simulink model "Human_in_Loop"  (R2017b)
settings: Solver=ode1  StartTime=0.0  StopTime=Inf  FixedStep=0.0002  RelTol=1e-3
PostLoadFcn:
  | , if any(exist('dsrtsu_mdlpostloadfcn', 'file') == [2, 3, 6]), try dsrtsu_mdlpostloadfcn('Execute', bdroot); catch fprintf('Error in PostLoadFcn (dsrtsu_mdlpostloadfcn) for model "%s":\n %s\n', bdroot, lasterr); end, end,
libraries: rti1202lib_dio_class1 x4, rti1202serlib x3, rtiemclib x2, rti1202lib_dac_class1 x1, simulink x1, rti1202lib_adc_class1 x1, rtitasklib x1
(part 2 of 2)

== system Human_in_Loop/Sensor Data/Cosmed/COSMED ==
  time : Inport
  count : Inport  Port=2
  DS1202SER_INT_C1_I1 : rti1202serlib/DS1202SER_INT_C1_I1  Reserved1=[]  Reserved2=[]  Reserved3=[]  Reserved4=[]  DSProperties=struct('RTI',struct('IOBoardType',{{'DS1202','SER'}},'SlaveProcessor','NONE','Version',uint32(3),'BlockType',struct('isSLSource',uint8(1),'isSLSink',uint8(0),'isHWSource',uint8(0),'isHWSink',uint8(0),'isSetup',uint8(0),'isInline',uint8(1),'isNonInline',uint8(0),'isInterrupt',uint8(1),'isChannelwise',uint8(1)),'UnitType','GENSER','Identifier','SERINT','DialogType','ML','BlockSet','NONE','RelationId',struct('TH',struct('BlockId','HWINT'))))  RTIBlockInterface=struct('BlockDisplay',{{['DS1202 SER Interrupt\n Channel 1\nReceive Interrupt'],'center'}},'BlockName',struct('Token',{{'DS1202SER_INT_C','_I'}},'BlockParam',{{'ChannelNo','IntType'}}),'OutputPortsWidth',int32(1),'OutputPortsActive',1,'OutputPortsName',{{[' ']}},'IconTransparency','off','ParameterTunableNames',{{}},'InitLevel',3,'DialogFcn','guigenserserint','MaskDescription',['To make the interrupts of the UART serial interface available as trigger source.'],'FunctionCall',uint32(0),'Options',{{'SS_OPTION_FORCE_NONINLINED_FCNCALL','SS_OPTION_ASYNCHRONOUS_INTERRUPT'}})  RTIBlockParameters=struct('ThIntNo',{{'UART_EVENTS','OFF',[]}},'ThSubIntNo',{{0,'ON',[0 4]}},'ThSrcSgnName',{{['UART Ch1 RX SW FIFO interrupt'],'OFF',[]}},'TLCFileName',{{'rti_hwinterrupt','OFF',[]}},'BoardNo',{{1,'ON',[1 1]}},'ChannelNo',{{1,'ON',[1 2]}},'ChannelNumOf',{{2,'OFF',[]}},'ThBlk',{{['struct(''blkh'',[''Human_in_Loop/Sensor Data/Cosmed/COSMED/DS1202SER_INT_C1_I1''],''srcId'',''UART_EVENTS_CH1_INT0'',''srcSgnId'',''UART_EVENTS_CH1_INT0'',''intervalTmrBlockId'',[],''srcSgnName'',[''UART Ch1 RX SW FIFO interrupt''],''srcCpuId'','''',''isSrcCpu'',1,''isTargetCpu'',1,''srcOnMasterCpu'',1,''boardType'','''',''boardTypeNo'','''',''boardNo'',1,''intNo'',''UART_EVENTS'',''subIntNo'',0,''period'',0,''entryPoint'',''rti_UART_EVENTS_CH1_INT0'',''blockName'',''DS1202SER_INT_C1_I1'',''taskNameDisplayExt'','''',''taskType'',''HWINT'',''groupId'',''SERINT'',''hookFcn'',''NULL'',''isTimerTaskSrc'',0,''service'','''',''mpBlkId'','''',''taskPriorityPreConfig'',''none'',''taskPriority'',-1,''taskSortWeighting'',[],''taskSchedulingPolicy'',''FCFS'',''taskOvrPreConfig'',''none'',''taskOvrStrategy'',1,''taskOvrQueueSize'',1,''taskVisibility'',''on'',''taskGroupId'','''',''taskGroupDisplayOrder'',[],''serviceDynamicGen'',0,''disableCodeGen'',0,''boardBase'',''IOLIB_SPEC_INT_UART(1)'',''noBoardBase'','''')'],'OFF',[]}},'IntType',{{1,'ON',[1 4]}},'ReceiveIntLevelFifo',{{'1','OFF',[]}},'IntTypeMacro',{{'DSSER_TRIGGER_LEVEL_SUBINT_MASK','OFF',[]}},'FifoSizeDefault',{{64,'OFF',[]}})  RTISFcnParameters=struct('BoardNo','double','ChannelNo','double','ThIntNo','double','ThSubIntNo','double','ThBlk','struct','IntType','double','ReceiveIntLevelFifo','double','TLCFileName','char','IntTypeMacro','char')  RTIBlockParaDefault=struct('ThIntNo',1,'ThSubIntNo',0,'ThSrcSgnName',['RX SW FIFO interrupt'],'TLCFileName','rti_hwinterrupt','BoardNo',1,'ChannelNo',1,'ChannelNumOf',2,'ThBlk',['struct(''srcSgnId'', '''')'],'IntType',1,'ReceiveIntLevelFifo',1,'IntTypeMacro','DSSER_TRIGGER_LEVEL_SUBINT_MASK','FifoSizeDefault',64)
  DS1202SER_SETUP_C1 : rti1202serlib/DS1202SER_SETUP_C1  Reserved1=[]  Reserved2=[]  Reserved3=[]  Reserved4=[]  DSProperties=struct('RTI',struct('Version',uint32(2),'IOBoardType',{{'DS1202','SER'}},'SlaveProcessor','NONE','BlockType',struct('isSLSource',uint8(0),'isSLSink',uint8(0),'isHWSource',uint8(0),'isHWSink',uint8(0),'isSetup',uint8(1),'isInline',uint8(1),'isNonInline',uint8(0),'isInterrupt',uint8(0),'isChannelwise',uint8(1)),'UnitType','GENSER','Identifier','SETUP','DialogType','ML','BlockSet','NONE'))  RTIBlockInterface=struct('BlockName',struct('Token',{{'DS1202SER_SETUP_C'}},'BlockParam',{{'ChannelNo'}}),'BlockDisplay',{{['Serial Setup'],'center'}},'IconTransparency','off','ParameterTunableNames',{{}},'InitLevel',1,'DialogFcn','guigensersetup','MaskDescription',['To set the global specifications for the UART interface.'])  RTIBlockParameters=struct('ParityMode',{{1,'OFF',[1 5]}},'TransceiverMode',{{[1;1],'OFF',[]}},'QuartzFrequency',{{'160000000','OFF',[]}},'BoardNo',{{1,'ON',[1 1]}},'ChannelNo',{{1,'ON',[1 2]}},'ChannelNumOf',{{2,'OFF',[]}},'BaudRate',{{'115200','OFF',[]}},'DataBitsNumOf',{{4,'OFF',[1 4]}},'StopBitsNumOf',{{1,'OFF',[1 3]}},'ReceiveIntLevelUart',{{4,'OFF',[1 4]}},'AutoflowMode',{{0,'OFF',[]}},'FifoSize',{{'256','OFF',[]}},'ReceiveIntLevelFifo',{{0,'OFF',[]}},'FifoOverrunMode',{{1,'OFF',[]}},'FifoBlockSize',{{'0','OFF',[]}},'TermMode',{{1,'OFF',[]}},'TLCFileName',{{'rtigensersetup','OFF',[]}})  RTISFcnParameters=struct('BoardNo','double','ChannelNo','double','ChannelNumOf','double','BaudRate','double','DataBitsNumOf','double','StopBitsNumOf','double','ParityMode','double','TransceiverMode','double','ReceiveIntLevelUart','double','AutoflowMode','double','FifoSize','double','ReceiveIntLevelFifo','double','FifoBlockSize','double','TermMode','double','QuartzFrequency','double','TLCFileName','char')  RTIBlockParaDefault=struct('ParityMode',1,'TransceiverMode',[1;1],'QuartzFrequency',160000000,'BoardNo',1,'ChannelNo',1,'ChannelNumOf',2,'BaudRate',115200,'DataBitsNumOf',4,'StopBitsNumOf',1,'ReceiveIntLevelUart',4,'AutoflowMode',0,'FifoSize',64,'ReceiveIntLevelFifo',0,'FifoOverrunMode',1,'FifoBlockSize',0,'TermMode',1,'TLCFileName','rtigensersetup')
  Serial Decoding System : Subsystem
  E : Outport
  wires:
  DS1202SER_INT_C1_I1/1 -> Serial Decoding System/Trigger
  Serial Decoding System/1(E) -> E/1
  time/1 -> Serial Decoding System/1(time)
  count/1 -> Serial Decoding System/2(count)

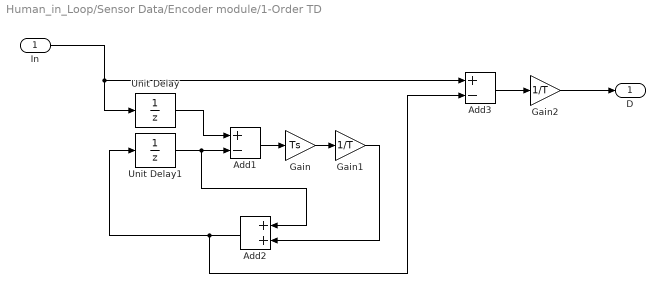
== system Human_in_Loop/Sensor Data/Encoder module/1-Order TD ==
  In : Inport
  Add1 : Sum  Inputs=+-
  Add2 : Sum
  Add3 : Sum  Inputs=+-
  Gain : Gain  Gain=Ts
  Gain1 : Gain  Gain=1/T
  Gain2 : Gain  Gain=1/T
  Unit Delay : UnitDelay  SampleTime=-1
  Unit Delay1 : UnitDelay  SampleTime=-1
  D : Outport
  wires:
  Unit Delay/1 -> Add1/1
  Add2/1 -> Add3/2, Unit Delay1/1
  Unit Delay1/1 -> Add2/1, Add1/2
  Add1/1 -> Gain/1
  Gain/1 -> Gain1/1
  Gain1/1 -> Add2/2
  In/1 -> Unit Delay/1, Add3/1
  Add3/1 -> Gain2/1
  Gain2/1 -> D/1

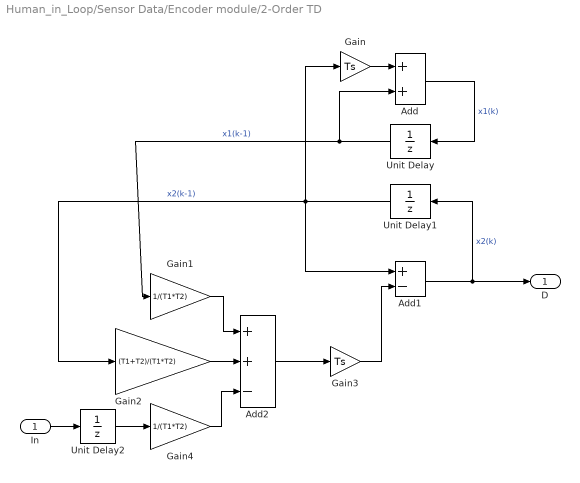
== system Human_in_Loop/Sensor Data/Encoder module/2-Order TD ==
  In : Inport
  Add : Sum
  Add1 : Sum  Inputs=+-
  Add2 : Sum  Inputs=++-
  Gain : Gain  Gain=Ts
  Gain1 : Gain  Gain=1/(T1*T2)
  Gain2 : Gain  Gain=(T1+T2)/(T1*T2)
  Gain3 : Gain  Gain=Ts
  Gain4 : Gain  Gain=1/(T1*T2)
  Unit Delay : UnitDelay  SampleTime=-1
  Unit Delay1 : UnitDelay  SampleTime=-1
  Unit Delay2 : UnitDelay  SampleTime=-1
  D : Outport
  wires:
  Unit Delay1/1 -> Gain2/1, Gain/1, Add1/1  "x2(k-1)"
  Gain/1 -> Add/1
  Add/1 -> Unit Delay/1  "x1(k)"
  Unit Delay/1 -> Gain1/1, Add/2  "x1(k-1)"
  Add1/1 -> D/1, Unit Delay1/1  "x2(k)"
  Gain1/1 -> Add2/1
  In/1 -> Unit Delay2/1
  Gain2/1 -> Add2/2
  Add2/1 -> Gain3/1
  Gain3/1 -> Add1/2
  Unit Delay2/1 -> Gain4/1
  Gain4/1 -> Add2/3

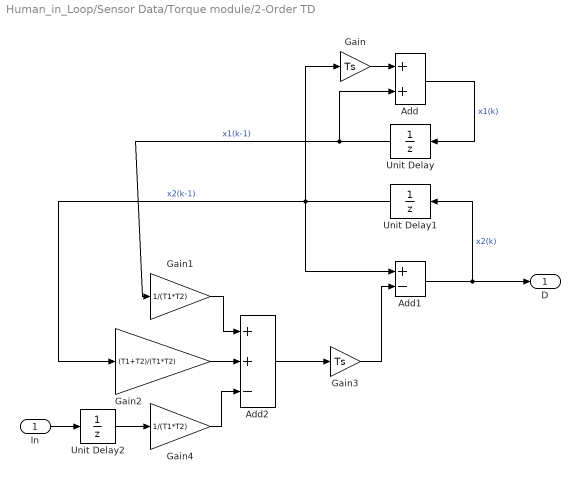
== system Human_in_Loop/Sensor Data/Torque module/2-Order TD ==
  In : Inport
  Add : Sum
  Add1 : Sum  Inputs=+-
  Add2 : Sum  Inputs=++-
  Gain : Gain  Gain=Ts
  Gain1 : Gain  Gain=1/(T1*T2)
  Gain2 : Gain  Gain=(T1+T2)/(T1*T2)
  Gain3 : Gain  Gain=Ts
  Gain4 : Gain  Gain=1/(T1*T2)
  Unit Delay : UnitDelay  SampleTime=-1
  Unit Delay1 : UnitDelay  SampleTime=-1
  Unit Delay2 : UnitDelay  SampleTime=-1
  D : Outport
  wires:
  Unit Delay1/1 -> Gain2/1, Gain/1, Add1/1  "x2(k-1)"
  Gain/1 -> Add/1
  Add/1 -> Unit Delay/1  "x1(k)"
  Unit Delay/1 -> Gain1/1, Add/2  "x1(k-1)"
  Add1/1 -> D/1, Unit Delay1/1  "x2(k)"
  Gain1/1 -> Add2/1
  In/1 -> Unit Delay2/1
  Gain2/1 -> Add2/2
  Add2/1 -> Gain3/1
  Gain3/1 -> Add1/2
  Unit Delay2/1 -> Gain4/1
  Gain4/1 -> Add2/3

== system Human_in_Loop/RTI Data/RTI Data Store/RTI Data Store/RTI Data Store ==
  RTI Data Store : Subsystem  mask(RTI_DATA_STORE){}
      mask help:
      | RTI Data Store Block. This block is used by RTI to store internal model dependent data. Deleting this block will result in data loss.
      |
      | NEVER DELETE, COPY, OR MODIFY THIS BLOCK!
      mask Help:
      | RTI Data Store Block. This block is used by RTI to store internal model dependent data. Deleting this block will result in data loss.
      | 
      | NEVER DELETE, COPY, OR MODIFY THIS BLOCK!
      mask Display: text(0.5, 0.5, ' ', 'HorizontalAlignment', 'center');

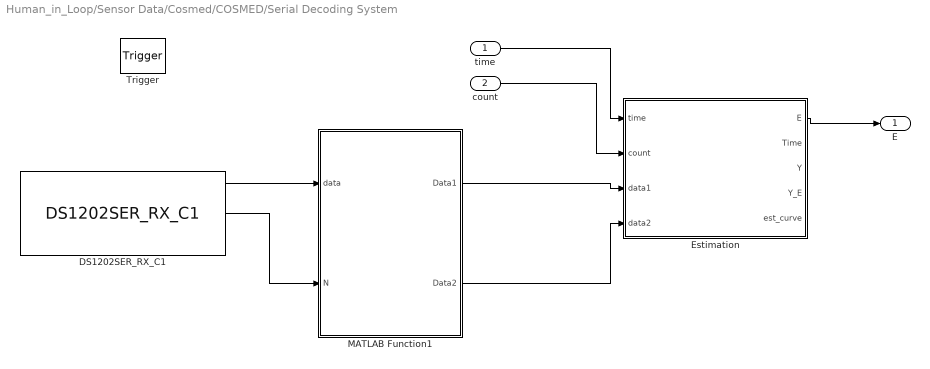
== system Human_in_Loop/Sensor Data/Cosmed/COSMED/Serial Decoding System ==
  time : Inport
  count : Inport  Port=2
  Trigger : TriggerPort  TriggerType=function-call  VariantControl=(inherit)
  DS1202SER_RX_C1 : rti1202serlib/DS1202SER_RX_C1  Reserved1=[]  Reserved2=[]  Reserved3=[]  Reserved4=[]  DSProperties=struct('RTI',struct('IOBoardType',{{'DS1202','SER'}},'SlaveProcessor','NONE','Version',uint32(1),'BlockType',struct('isSLSource',uint8(1),'isSLSink',uint8(1),'isHWSource',uint8(0),'isHWSink',uint8(1),'isSetup',uint8(0),'isInline',uint8(1),'isNonInline',uint8(0),'isInterrupt',uint8(0),'isChannelwise',uint8(1)),'UnitType','GENSER','Identifier','RECEIVE','DialogType','ML','BlockSet','NONE'))  RTIBlockInterface=struct('BlockName',struct('Token',{{'DS1202SER_RX_C'}},'BlockParam',{{'ChannelNo'}}),'InputPortsWidth',int32(1),'InputPortsActive',0,'InputPortsDataType',{{'SS_UINT32'}},'InputPortsName',{{'NumBytes'}},'OutputPortsWidth',int32([16 1 1]),'OutputPortsActive',[1 1 1],'OutputPortsDataType',{{'SS_UINT8','SS_UINT32','SS_INT32'}},'OutputPortsName',{{'RXBytes','NumRXBytes','Status'}},'BlockDisplay',{{['Serial Receive'],'center'}},'IconTransparency','on','ParameterTunableNames',{{}},'InitLevel',2,'DialogFcn','guigenserreceive','MaskDescription',['To read data from the UART SW FIFO.'])  RTIBlockParameters=struct('BoardNo',{{1,'ON',[1 1]}},'ChannelNo',{{1,'ON',[1 2]}},'ChannelNumOf',{{2,'OFF',[]}},'ReceptionDataMode',{{1,'OFF',[]}},'ParamTunableMode',{{2,'OFF',[]}},'BytesRefNumOfT',{{'1','OFF',[1 inf]}},'BytesRefNumOfNT',{{'16','OFF',[1 inf]}},'BytesRefNumOfMax',{{'1','OFF',[1 inf]}},'BytesRefNumOfMode',{{0,'OFF',[]}},'BytesActNumOfMode',{{1,'OFF',[]}},'ReceptionStatusMode',{{1,'OFF',[]}},'FifoSizeDefault',{{64,'OFF',[]}},'TLCFileName',{{'rtigenserreceive','OFF',[]}})  RTISFcnParameters=struct('BoardNo','double','ChannelNo','double','ChannelNumOf','double','ReceptionDataMode','double','ParamTunableMode','double','BytesRefNumOfT','double','BytesRefNumOfNT','double','BytesRefNumOfMax','double','BytesRefNumOfMode','double','BytesActNumOfMode','double','ReceptionStatusMode','double','TLCFileName','char')  RTIBlockParaDefault=struct('BoardNo',1,'ChannelNo',1,'ChannelNumOf',2,'ReceptionDataMode',1,'ParamTunableMode',1,'BytesRefNumOfT',1,'BytesRefNumOfNT',1,'BytesRefNumOfMax',1,'BytesRefNumOfMode',0,'BytesActNumOfMode',1,'ReceptionStatusMode',1,'FifoSizeDefault',64,'TLCFileName','rtigenserreceive')
  Estimation : MATLAB Function  TreatAsAtomicUnit=on
  MATLAB Function1 : MATLAB Function  TreatAsAtomicUnit=on
  E : Outport
  wires:
  DS1202SER_RX_C1/2 -> MATLAB Function1/2(N)
  MATLAB Function1/1(Data1) -> Estimation/3(data1)
  DS1202SER_RX_C1/1 -> MATLAB Function1/1(data)
  time/1 -> Estimation/1(time)
  count/1 -> Estimation/2(count)
  Estimation/1(E) -> E/1
  MATLAB Function1/2(Data2) -> Estimation/4(data2)

== system Human_in_Loop/RTI Data/RTI Data Store/RTI Data Store/RTI Data Store/RTI Data Store ==

== matlab function Human_in_Loop/Sensor Data/Encoder module/Data process ==
  data: encoder input; angle output; BT_RESET_ANKLE parameter boolean
function angle = process(encoder, BT_RESET_ANKLE)

    persistent angle_zero;
    if isempty(angle_zero)
        angle_zero = 0;
    end

    if BT_RESET_ANKLE == 1
        angle_zero = encoder;
    end

    angle = encoder - angle_zero;
end

== matlab function Human_in_Loop/Sensor Data/Encoder module/Data process1 ==
  data: encoder input; BT_RESET_MOTOR parameter boolean; angle output
function angle = process(encoder, BT_RESET_MOTOR)

    persistent angle_zero;
    if isempty(angle_zero)
        angle_zero = 0;
    end

    if BT_RESET_MOTOR == 1
        angle_zero = encoder;
    end

    angle = encoder - angle_zero;
    
end

== matlab function Human_in_Loop/Sensor Data/Encoder module/Mux ==
  data: x1 input; x output; x2 input
function x = mux(x1,x2)

x = [x1 x2];

== matlab function Human_in_Loop/Sensor Data/Torque module/Data process ==
  data: vol input; torque output; load_vol_gain parameter double; load_vol_offset parameter double; BT_RESET_TORQUE parameter boolean
function torque = process(vol, load_vol_gain, load_vol_offset, BT_RESET_TORQUE)
%% 功能：电压-力矩转换与力矩归零

    persistent torque_zero;
    if isempty(torque_zero)
        torque_zero = 0;
    end

    %%% 力矩归零
    if BT_RESET_TORQUE == 1
        torque_zero = vol*load_vol_gain + load_vol_offset;
    end

    torque = vol*load_vol_gain + load_vol_offset - torque_zero;

end

== matlab function Human_in_Loop/Sensor Data/Encoder module/Mux1 ==
  data: x1 input; x output; x2 input; x3 input
function x = mux(x1,x2,x3)

x = [x1 x2 x3];

== matlab function Human_in_Loop/Sensor Data/Encoder module/Mux2 ==
  data: x1 input; x output; x2 input; x3 input
function x = mux(x1,x2,x3)

x = [x1 x2 x3];

== matlab function Human_in_Loop/Sensor Data/FootSwitch module/FootSwitch Filter ==
  data: signal input; state output
function state = filter(signal)

%% 对足底开关信号进行滤波
% 滤波原则：上升沿无滤波，下降沿消抖滤波

Ts = 0.0002;
persistent foot_state;
persistent filter_time;
if isempty(foot_state)
    foot_state = 0;
    filter_time = 0;
end

if foot_state == 0
    if signal == 1
        foot_state = 1;
    else
        foot_state = 0;
    end
else
    if signal == 1
        foot_state = 1;
    else
        filter_time = filter_time + Ts;
        if filter_time > 0.1
            filter_time = 0;
            foot_state = 0;
        end
    end
end
   
state = foot_state;

end

== matlab function Human_in_Loop/Parameter Module/Control Parameter/Mux1 ==
  data: x1 input; x output; x2 input; x3 input; x4 input; x5 input
function x = mux(x1,x2,x3,x4,x5)

x = [x1 x2 x3 x4 x5];

== matlab function Human_in_Loop/Parameter Module/Torque Parameter/Mux1 ==
  data: x1 input; x output; x2 input; x3 input; x4 input
function x = mux(x1,x2,x3,x4)

x = [x1 x2 x3,x4];

== matlab function Human_in_Loop/State Module/State Machine ==
  data: mode output; footswitch input; state output; BT_RUN parameter boolean; BT_SLACK parameter boolean; BT_IDLE parameter boolean; BT_ERROR parameter boolean; stride_time output; BT_CALIB parameter boolean; stride_timer output
function [mode,state,stride_time,stride_timer] = StateMechine(footswitch, BT_RUN, BT_SLACK, BT_IDLE, BT_ERROR, BT_CALIB)

%% 定义寄存变量
persistent reg_stride_time;
persistent reg_stride_time_count;
persistent reg_mode;
persistent reg_state;
persistent bt_run;
persistent reg_last_switch;
if isempty(reg_stride_time)
    reg_stride_time = 1;
    reg_stride_time_count = 0;
    reg_mode = 1;
    reg_state = 1;
    bt_run = 0;
    reg_last_switch = 1;
end

%% 参数定义
Ts = 0.0002;
PP_StandSwing = 0.6;
max_stride_time = 1.5;
min_sride_time = 0.5;

%% 模式说明
IDLE_MODE  = 1;
RUN_MODE   = 2;
SLACK_MODE = 3;
CALIB_MODE = 4;
ERROR_MODE = 0;

%% 模式转换
if BT_RUN == 1
    bt_run = 1;
end
if BT_CALIB == 1
    reg_mode = CALIB_MODE;
end
if BT_SLACK == 1
    reg_mode = SLACK_MODE;
end
if BT_IDLE == 1
    reg_mode = IDLE_MODE;
end
if BT_ERROR == 1
    reg_mode = ERROR_MODE;
end
% 运行模式在swing->stance时切换
if bt_run == 1 && reg_last_switch == 0 && footswitch == 1
    reg_mode = RUN_MODE;
    bt_run = 0;
end
        
if reg_mode == RUN_MODE || reg_mode == IDLE_MODE
    if reg_last_switch == 0 && footswitch == 1
        reg_state = 1;
        reg_stride_time = 0.618*reg_stride_time + 0.382*reg_stride_time_count;
        reg_stride_time_count = 0;
    elseif reg_state ==1 && reg_stride_time_count > PP_StandSwing * reg_stride_time
        reg_state = 0;
        reg_stride_time_count = reg_stride_time_count + Ts;
    else
        reg_stride_time_count = reg_stride_time_count + Ts;
    end
end

reg_last_switch = footswitch;
if reg_stride_time > max_stride_time
    reg_stride_time = max_stride_time;
elseif reg_stride_time < min_sride_time
    reg_stride_time = min_sride_time;
end

mode = reg_mode;
state = reg_state;
stride_time = reg_stride_time;
stride_timer = reg_stride_time_count;

end

== matlab function Human_in_Loop/State Module/Mux1 ==
  data: x1 input; x output; x2 input; x3 input; x4 input
function x = mux(x1,x2,x3,x4)

x = [x1 x2 x3,x4];

== matlab function Human_in_Loop/Control Module/Controller ==
  data: state input; motor_vel_cmd output; torque input; ankle input; motor input; control_parm input; torque_trace_des input; torque_delta_trace_des input; lrn_cmd input; run_mode parameter int8; CALIB_TORQUE parameter double; CALIB_SPEED parameter double; SLACK_SPEED parameter double; FOLLOW_SLACK_ANGLE parameter double; TorqueMem data_store_memory; SWING_MAX_ANGLE parameter double
function motor_vel_cmd  = control(state,torque,ankle,motor,control_parm,torque_trace_des,torque_delta_trace_des,lrn_cmd, run_mode,CALIB_TORQUE,CALIB_SPEED, SLACK_SPEED,FOLLOW_SLACK_ANGLE,SWING_MAX_ANGLE)

%% 寄存变量声明
persistent calib_state;
if isempty(calib_state)
    calib_state = 0;
end

%% 模式定义
IDLE_MODE  = 1;
RUN_MODE   = 2;
SLACK_MODE = 3;
CALIB_MODE = 4;
ERROR_MODE = 0;

%% 控制模式定义
FOLLOW_MODE = 1;
TORQUE_MODE = 2;

%% 参数定义
GearRatio = 5;
RadiusRatio = 40/120;
MotorTimeConstance = 0.05;

%% 数据提取
mode = state(1);
footstate = state(2);
stride_time = state(3);
stride_timer = state(4);

ankle_angle = ankle(1);
ankle_gyro = ankle(2);
motor_angle = motor(1);
motor_gyro = motor(2);

torque_measure = torque(1);
torque_delta = torque(2);
torque_des = torque_trace_des;
torque_delta_des = torque_delta_trace_des;

Kp = control_parm(1);
Kd = control_parm(2);
Ks = control_parm(4);
Ko = control_parm(5);

switch mode
    case IDLE_MODE
        motor_vel_cmd = 0;
        calib_state = 0;
        
    case SLACK_MODE
        motor_vel_cmd = -SLACK_SPEED*GearRatio;
        
    case CALIB_MODE
        if calib_state == 0 && torque_measure < CALIB_TORQUE
            motor_vel_cmd = CALIB_SPEED*GearRatio;
        elseif calib_state == 0 && torque_measure > CALIB_TORQUE
            calib_state = 1;
            motor_vel_cmd = 0;
        else
            motor_vel_cmd = 0;
        end
        
    case RUN_MODE
        switch run_mode
            
            case FOLLOW_MODE
                if ankle_angle > 0
                    angle_error = ankle_angle - (ankle_angle/50)*FOLLOW_SLACK_ANGLE - motor_angle*RadiusRatio;
                else 
                    angle_error = ankle_angle - motor_angle*RadiusRatio;
                end
                motor_vel_cmd = Ks*angle_error*GearRatio/MotorTimeConstance;
                
            case TORQUE_MODE
                if footstate == 1
                    torque_error = torque_des - torque_measure;
                    torque_delta_error = torque_delta_des - torque_delta;
                    speed_des = Ko*torque_delta_des;
                    motor_vel_cmd = (Kp*torque_error + Kd*torque_delta_error + lrn_cmd + speed_des) * GearRatio / MotorTimeConstance;
                else
                    angle_error = 0 - motor_angle*RadiusRatio;
                    motor_vel_cmd = ( Ks * angle_error ) * GearRatio / MotorTimeConstance;
                end
            otherwise
                motor_vel_cmd = 0;
        end
        
    case ERROR_MODE
        motor_vel_cmd = 0;
        
    otherwise
        motor_vel_cmd = 0;
end


end

== matlab function Human_in_Loop/Control Module/Motor/MATLAB Function ==
  data: torque input; vel output; ankle input; motor input; motor_vel_cmd input; MAX_TORQUE parameter double; MAX_MOTOR_ANGLE parameter double; MIN_MOTOR_ANGLE parameter double; MAX_SPEED parameter double
function vel = fcn(torque,ankle,motor,motor_vel_cmd,MAX_TORQUE, MAX_MOTOR_ANGLE, MIN_MOTOR_ANGLE, MAX_SPEED)

motor_angle = motor(1);
torque_measure = torque(1);

if torque_measure > MAX_TORQUE
    vel = 0;
elseif motor_angle > MAX_MOTOR_ANGLE
    vel = 0;
elseif motor_angle < MIN_MOTOR_ANGLE
    vel = 0;
elseif motor_vel_cmd > MAX_SPEED
    vel = MAX_SPEED;
elseif motor_vel_cmd < - MAX_SPEED
    vel = - MAX_SPEED;
else
    vel = motor_vel_cmd;
end

end

== matlab function Human_in_Loop/Control Module/Torque track ==
  data: torque_parm input; torque input; torque_des output; torque_delta_des output; state input; TorqueMem data_store_memory; torque_trace output; torque_delta_trace output
function [torque_des,torque_delta_des,torque_trace,torque_delta_trace] = TorqueTrack(torque_parm,torque,state)

%% 寄存变量声明
global TorqueMem;

persistent last_footstate;
if isempty(last_footstate)
    last_footstate = 0;
end

%% 参数定义
Fs = 500;

%% 模式定义
IDLE_MODE  = 1;
RUN_MODE   = 2;

%% 数据提取
mode = state(1);
footstate = state(2);
stride_time = state(3);
stride_timer = state(4);

peak_torque = torque_parm(1);
rise_time = torque_parm(2);
peak_time = torque_parm(3);
fall_time = torque_parm(4);

torque_measure = torque(1);
troque_delta = torque(2);
stride_index = stride_timer*Fs + 1;
if stride_index > 750
    stride_index = 750;
end

%% 更新期望力矩曲线
if last_footstate == 0 && footstate == 1 && (mode == RUN_MODE || mode == IDLE_MODE)
    
    torque_track = zeros(1,750);
    torque_delta_track = zeros(1,750);
    time_index = 1:750;
    one_line = ones(1,750);
    index_peak = floor(peak_time/100*stride_time*Fs);
    index_rise = index_peak - floor(rise_time/100*stride_time*Fs);
    index_fall = index_peak + floor(fall_time/100*stride_time*Fs);
    
    % 构造三次样条函数方程组
    A1 = [1,index_rise,index_rise^2,index_rise^3;
          1,index_peak,index_peak^2,index_peak^3;
          0,1,2*index_rise,3*index_rise^2;
          0,1,2*index_peak,3*index_peak^2];
    b1 = [0;peak_torque;0;0];
    parm1 = (A1\b1)';
    torque_track(floor(index_rise):floor(index_peak-1)) = parm1*[one_line(1:floor(index_peak-index_rise));time_index(floor(index_rise):floor(index_peak-1));time_index(floor(index_rise):floor(index_peak-1)).^2;time_index(floor(index_rise):floor(index_peak-1)).^3];
    torque_delta_track(index_rise:index_peak-1) = parm1(2:4)*[one_line(1:index_peak-index_rise);2*time_index(index_rise:index_peak-1);3*time_index(index_rise:index_peak-1).^2]*Fs;
    
    A2 = [1,index_peak,index_peak^2,index_peak^3;
          1,index_fall,index_fall^2,index_fall^3;
          0,1,2*index_peak,3*index_peak^2;
          0,1,2*index_fall,3*index_fall^2];
    b2 = [peak_torque;0;0;0];
    parm2 = (A2\b2)';
    torque_track(floor(index_peak):floor(index_fall)) = parm2*[one_line(1:floor(index_fall+1-index_peak));time_index(floor(index_peak):floor(index_fall));time_index(floor(index_peak):floor(index_fall)).^2;time_index(floor(index_peak):floor(index_fall)).^3];
    %注释此处代码，考虑了力矩上升与下降的非线性
    %torque_delta_track(index_peak:index_fall) = parm2(2:4)*[one_line(1:index_fall+1-index_peak);2*time_index(index_peak:index_fall);3*time_index(index_peak:index_fall).^2]*Fs/2;
    
    TorqueMem(1,1:750) = torque_track(1:750);
    %TorqueMem(2,1:750) = zeros(1,750);
    TorqueMem(3,1:750) = torque_delta_track(1:750);
    %TorqueMem(4,1:750) = zeros(1,750);
end

last_footstate = footstate;
TorqueMem(2,stride_index) = torque_measure;
TorqueMem(4,stride_index) = troque_delta;

if mode == RUN_MODE
    torque_des = TorqueMem(1,stride_index);
    torque_delta_des = TorqueMem(3,stride_index);
else
    torque_des = 0;
    torque_delta_des = 0;
end

torque_trace = TorqueMem(1:2,1:750);
torque_delta_trace = TorqueMem(3:4,1:750);

end

== matlab function Human_in_Loop/Control Module/LRN ==
  data: lrn_cmd output; state input; control_parm input; BT_LRN_CLEAR parameter boolean; BT_LRN_ON parameter boolean; error_filter_k parameter double; time_delay parameter int32; lrn_mem output; TorqueMem data_store_memory; lrn_shrink parameter double
function [lrn_cmd, lrn_mem] = LRN_controller(state,control_parm, BT_LRN_CLEAR, BT_LRN_ON, error_filter_k, time_delay, lrn_shrink)

global TorqueMem;

persistent last_footstate;
persistent torque_error_memory;
persistent lrn_cmd_memory;
if isempty(last_footstate)
    last_footstate = 0;
    torque_error_memory = zeros(1,1000);
    lrn_cmd_memory = zeros(1,1000);
end

%% 参数定义
Fs = 500;

%% 模式定义
IDLE_MODE  = 1;
RUN_MODE   = 2;

%% 数据提取
mode = state(1);
footstate = state(2);
stride_time = state(3);
stride_timer = state(4);

Kl = control_parm(3);

stride_index = stride_timer*Fs + 1;
if stride_index > 750
    stride_index = 750;
end

if last_footstate == 0 && footstate == 1 && mode == RUN_MODE && BT_LRN_ON == 1
    error = TorqueMem(1,1:750) - TorqueMem(2,1:750);
    torque_error_memory(1:750) = (1-error_filter_k)*torque_error_memory(1:750) + error_filter_k*error;
    lrn_cmd_memory(1:750) = lrn_shrink*lrn_cmd_memory(1:750) + Kl*torque_error_memory(1:750);
end

if BT_LRN_CLEAR == 1
    torque_error_memory = zeros(1,1000);
    lrn_cmd_memory = zeros(1,1000);
end

if mode == RUN_MODE
    if stride_index >= 750 - floor(time_delay)
        lrn_cmd = 0;
    else
        lrn_cmd = lrn_cmd_memory(1,stride_index + floor(time_delay));
    end
else
    lrn_cmd = 0;
end

last_footstate = footstate;
lrn_mem = lrn_cmd_memory(1:750);


end

== matlab function Human_in_Loop/Sensor Data/Cosmed/COSMED/Serial Decoding System/Estimation ==
  data: time input; E output; count input; data1 input; Time output; Y output; data2 input; Y_E output; est_curve output
function [E,Time,Y,Y_E,est_curve] = Estimation(time,count,data1,data2)

%% 定义状态变量与参数常量
persistent last_count;  %上次Timer周期
persistent x;           %最小二乘的自变量（x = 1-exp（t/T））
persistent y;           %最小二乘的因变量（y = data）
persistent theta;       %最小二乘计算的参数
persistent num;         %离散数据点的个数
T = 42;

%% 状态变量初始化
if isempty(last_count)
    last_count = -1;
    x = [10:10:200];
    y = zeros(1,20);
    theta = zeros(2,1);
    num = 1;
end

%% 判断新周期与更新num
if last_count ~= count || count == 0
    last_count = count;
    x = 10:10:200;
    y = zeros(1,20);
    theta = zeros(2,1);
    num = 1;
else
    num = num + 1;
end

%% 数据记录
if count ~= 0
    x(num) = time;
    y(num) = 0.278*data1 + 0.075*data2;

    %% 参数最小二乘辨识
    if num >= 2
        A = [(1-exp(-x(1:num)'/T)),ones(num,1)];
        b = y(1:num)';
        theta = A\b;
    end
end

%% 结果输出
E = theta(1)+theta(2);

Time = x(1:12);
Y = y(1:12);
Y_E = ([(1-exp(-Time'./T)),ones(12,1)]*theta(1:2))';
est_curve = [Y;Y_E];

== matlab function Human_in_Loop/Sensor Data/Torque module/Mux ==
  data: x1 input; x output; x2 input
function x = mux(x1,x2)

x = [x1 x2];

== matlab function Human_in_Loop/Sensor Data/Cosmed/COSMED/Serial Decoding System/MATLAB Function1 ==
  data: data input; N input; Data1 output double; Data2 output
function [Data1,Data2]  = Decoder(data,N)

Data1 = 0;
Data2 = 0;

i = 1;

while data(i) ~= ','
    Data1 = Data1*10 + (double(data(i))-48);
    i = i + 1;
end

i = i + 1;

while i < N
    Data2 = Data2*10 + (double(data(i))-48);
    i = i + 1;
end

end

== matlab function Human_in_Loop/Sensor Data/Torque module/MATLAB Function ==
  data: torque input; torque_dot output
function torque_dot = fcn(torque)

persistent data;
if isempty(data)
    data = ones(15,1);
end

data = [data(2:15);torque];

a1 = ones(15,1);
a2 = (1:15)';
A = [a1 a2];
x = A\data;

torque_dot = x(2)*5000;

== matlab function Human_in_Loop/Sensor Data/Cosmed/Timer ==
  data: Trigger output; Time output; Count output; BT_METAB_EST parameter boolean
function [Trigger, Time, Count] = Timer(BT_METAB_EST)

persistent tigger;
persistent count;
persistent time;

Ts = 0.0002;     %采样时间
T_L = 120;        %间隔时间

if isempty(tigger)
    tigger = 0;
    count = 0;
    time = 0;
end

if BT_METAB_EST == 1
    if(time > T_L)
        time = 0;
        count = count + 1;
        tigger = 1;
    else
        time  = time + Ts;
        tigger = 0;
    end
else
    tigger = 0;
    count = 0;
    time = time + Ts;
end

Trigger = tigger;
Time = time;
Count = count;
